simulink library "sf_gui_elevator_controller_lib"  (R2017b)
settings: Solver=FixedStepDiscrete  StartTime=0.0  StopTime=10.0  FixedStep=1  RelTol=1e-3  EnableMultiTasking=on
settings Model: Creator=The MathWorks, Inc.  LastModifiedBy=The MathWorks, Inc.
settings DataIOCC: LimitDataPoints=on  SaveFormat=Array  SignalLoggingSaveFormat=ModelDataLogs
settings OptimizationCC: ExpressionDepthLimit=2147483647  LifeSpan=inf
settings DebuggingCC: UnderspecifiedInitializationDetection=Classic  MergeDetectMultiDrivingBlocksExec=none  SolverPrmCheckMsg=warning  FcnCallInpInsideContextMsg=warning  StateNameClashWarn=warning  SFUnexpectedBacktrackingDiag=warning  SFNoUnconditionalDefaultTransitionDiag=warning  SFExecutionAtInitializationDiag=none
settings HardwareCC: ProdBitPerPointer=32  ProdBitPerSizeT=32  ProdBitPerPtrDiffT=32  ProdLargestAtomicFloat=None  ProdIntDivRoundTo=Undefined  ProdEndianess=Unspecified  ProdWordSize=32  ProdHWDeviceType=32-bit Generic
settings ModelReferenceCC: PropagateSignalLabelsOutOfModel=off
settings CodeAppCC: StateflowObjectComments=on
settings GRTTargetCC: TargetLangStandard=C89/C90 (ANSI)  GeneratePreprocessorConditionals=Disable all  CombineOutputUpdateFcns=off  GRTInterface=on
settings ConfigComp: CovMetricSettings=dw  CovHtmlReporting=on  CovSaveCumulativeToWorkspaceVar=on  CovSaveSingleToWorkspaceVar=on  CovExternalEMLEnable=off

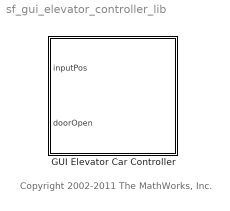
== system sf_gui_elevator_controller_lib ==
  note: Copyright 2002-2011 The MathWorks, Inc.
  GUI Elevator Car Controller : Stateflow chart  TreatAsAtomicUnit=on

== stateflow chart sf_gui_elevator_controller_lib/GUI Elevator Car Controller ==
  state Controller
    state close_door [function]
      (default) -> (junction 58) : {ml.sf_elevator_gui('close_door', carID);}
    state open_door [function]
      (default) -> (junction 55) : {ml.sf_elevator_gui('open_door', carID);}
    state move(pos) [function]
      (default) -> (junction 61) : {ml.sf_elevator_gui('move_car', carID, pos);}
    state deactivate_hall_button(pos) [function]
      (default) -> (junction 89) : {ml.sf_elevator_gui('deactivate', 'hall', get_floor_number(pos));}
    state deactivate_car_button(pos) [function]
      (default) -> (junction 74) : {floorNum = get_floor_number(pos);
          | ml.sf_elevator_gui('deactivate',carID, floorNum);}
    state floorNumber = get_floor_number(pos) [function]
      (default) -> (junction 79) : {floorNumber = ml.round(pos);}
    Controller -> (junction 2)
    (junction 2) -> (junction 3) [order 1] : [hasChanged(inputPos)]
    (junction 2) -> (junction 4) [order 2]
    (junction 3) -> (junction 5) : {move(inputPos);}
    (junction 5) -> (junction 4)
    (junction 4) -> (junction 6)
    (junction 6) -> (junction 7) [order 1] : [hasChanged(doorOpen)]
    (junction 6) -> (junction 10) [order 2]
    (junction 7) -> (junction 8)
    (junction 8) -> (junction 9) [order 1] : [doorOpen]
    (junction 8) -> (junction 11) [order 2] : {close_door();}
    (junction 9) -> (junction 12) : {open_door();}
    (junction 11) -> (junction 10) : {deactivate_hall_button(inputPos);
        |  deactivate_car_button(inputPos);}
    (junction 12) -> (junction 11)
    (junction 10) -> (junction 13)
  data: pos function_input double; pos function_input double; pos function_input double; floorNum temporary double; pos function_input double; floorNumber function_output double; inputPos input; doorOpen input; carID parameter
